simulink model "TestPID"  (R2022a)
settings: Solver=VariableStepAuto  StartTime=0.0  StopTime=10.0  RelTol=1e-3
values from neighbouring files (symbols this model uses):
  a_theta1 = den(2)    [computeGains.m]    (also in compute_tf_model.m = -rho*Va_trim^2*cbar*S_wing/2/P.Jy*C_M_q*cbar/2/Va_trim)
  a_theta2 = den(3)    [computeGains.m]    (also in compute_tf_model.m = -rho*Va_trim^2*cbar*S_wing/2/P.Jy*C_M_alpha)
  a_theta3 = num(3)    [computeGains.m]    (also in compute_tf_model.m = rho*Va_trim^2*cbar*S_wing/2/P.Jy*C_M_delta_e)
undefined symbols (not defined in the file or in its folder): P
settings Model: Creator=berka  LastModifiedBy=berka

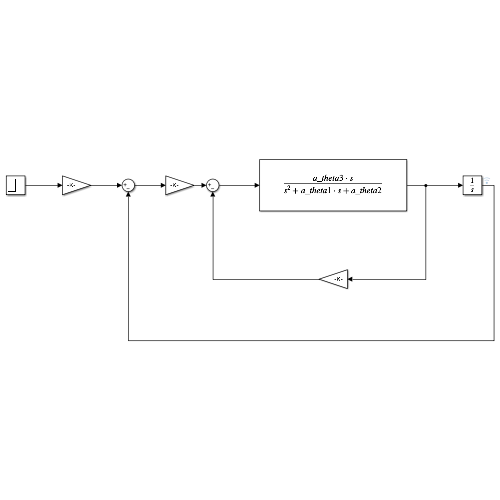
[thumbnail: Simulink's stored preview of the top-level diagram]
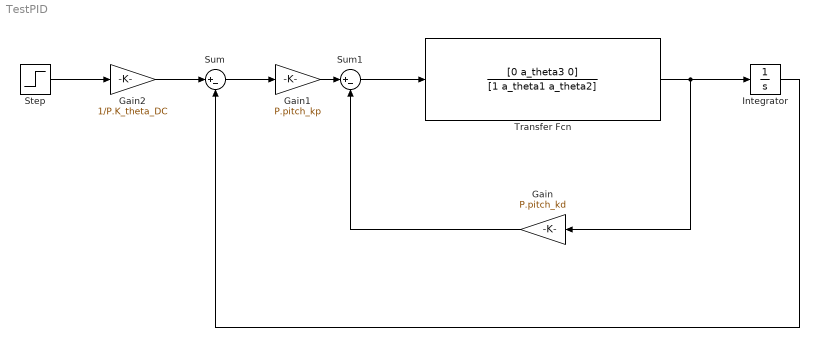
== system TestPID ==
  Gain : Gain  Gain=P.pitch_kd
  Gain1 : Gain  Gain=P.pitch_kp
  Gain2 : Gain  Gain=1/P.K_theta_DC
  Integrator : Integrator
  Step : Step  SampleTime=0
  Sum : Sum  Inputs=|+-
  Sum1 : Sum  Inputs=|+-
  Transfer Fcn : TransferFcn  Numerator=[0 a_theta3 0]  Denominator=[1 a_theta1 a_theta2]
  wires:
  Transfer Fcn/1 -> Integrator/1, Gain/1
  Gain/1 -> Sum1/2
  Sum/1 -> Gain1/1
  Gain1/1 -> Sum1/1
  Integrator/1 -> Sum/2
  Sum1/1 -> Transfer Fcn/1
  Step/1 -> Gain2/1
  Gain2/1 -> Sum/1
